simulink model "LatchHandler"  (R2016b)
settings: Solver=VariableStepAuto  StartTime=0.0  StopTime=10.0  RelTol=1e-3
settings Model: Creator=Nathan  LastModifiedBy=Nathan

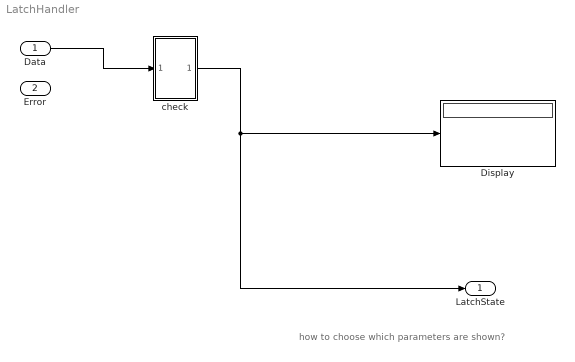
== system LatchHandler ==
  note: how to choose which parameters are shown?
  Data : Inport
  Error : Inport  Port=2
  Display : Display
  check : Subsystem
  LatchState : Outport
  wires:
  check/1(Out1) -> Display/1, LatchState/1
  Data/1 -> check/1(In1)

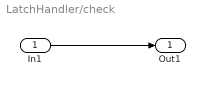
== system LatchHandler/check ==
  In1 : Inport
  Out1 : Outport
  wires:
  In1/1 -> Out1/1
